simulink model "LAB07_1_copia2"  (R2022b)
settings: Solver=ode8  StartTime=0.0  StopTime=1000  FixedStep=0.1  RelTol=1e-3
values from neighbouring files (symbols this model uses):
  a = 6.843e6    (= 6843000)    [LAB_07_script.m]    (also in LAB_07_with3Dplot.m)
  A0 = eye(3,3)    [LAB_07_script.m]    (also in LAB_07_with3Dplot.m)
  A1 = 0.02    [LAB_07_with3Dplot.m]
  A2 = A1    (= 0.02)    [LAB_07_with3Dplot.m]
  A3 = A1    (= 0.02)    [LAB_07_with3Dplot.m]
  alpha_1 = 0.5    [LAB_07_with3Dplot.m]
  alpha_2 = 0.5    [LAB_07_with3Dplot.m]
  C_d = 2.1    [LAB_07_with3Dplot.m]
  e = 0    [LAB_07_script.m]    (also in LAB_07_with3Dplot.m)
  epsilon = 0.4093    [LAB_07_script.m]    (also in LAB_07_with3Dplot.m)
  G = 6.6743e-11    [LAB_07_script.m]    (also in LAB_07_with3Dplot.m)
  g_01 = -29404.8    [LAB_07_script.m]    (also in LAB_07_with3Dplot.m)
  g_11 = -1450.9    [LAB_07_script.m]    (also in LAB_07_with3Dplot.m)
  h_11 = 4652.5    [LAB_07_script.m]    (also in LAB_07_with3Dplot.m)
  i = 0.1    [LAB_07_script.m]    (also in LAB_07_with3Dplot.m)
  I = 10^-2*diag([100.9,25.1,91.6])    [LAB_07_script.m]    (also in LAB_07_with3Dplot.m)
  j_B = [0.01;0.05;0.01]    [LAB_07_script.m]    (also in LAB_07_with3Dplot.m)
  M_Earth = 5.972e24    (= 5.972e+24)    [LAB_07_script.m]    (also in LAB_07_with3Dplot.m)
  n = sqrt(G*M_Earth/a^3)    [LAB_07_script.m]    (also in LAB_07_with3Dplot.m)
  n_sun = 2*pi/T_sun    (= 1.99238499086e-07)    [LAB_07_script.m]    (also in LAB_07_with3Dplot.m)
  P = F_e/c    (= 4.52666666667e-06)    [LAB_07_script.m]    (also in LAB_07_with3Dplot.m)
  position = 1e-2*[10,0,0;0,10,0;-10,0,0;0,-10,0;0,0,15;                                     0,0,-15;0,45,0;0,45,0;0,-45,0;0,-45,0]    [LAB_07_script.m]    (also in LAB_07_with3Dplot.m)
  R_Earth = 6.378e6    (= 6378000)    [LAB_07_script.m]    (also in LAB_07_with3Dplot.m)
  R_sun = 149597870000    [LAB_07_script.m]    (also in LAB_07_with3Dplot.m)
  rhoD_vector = ones(10,1)*0.1    [LAB_07_script.m]    (also in LAB_07_with3Dplot.m)
  rhoS_vector = ones(10,1)*0.5    [LAB_07_script.m]    (also in LAB_07_with3Dplot.m)
  Surfaces_Matrix = [6e-2;6e-2;6e-2;6e-2;4e-2;4e-2;12e-2;                                                     12e-2;12e-2;12e-2]    [LAB_07_script.m]    (also in LAB_07_with3Dplot.m)
  theta0 = 0    [LAB_07_script.m]    (also in LAB_07_with3Dplot.m)
  Theta_m = deg2rad(11.5)    [LAB_07_script.m]    (also in LAB_07_with3Dplot.m)
  Versor_Surfaces_Matrix = [  1 , 0 ,-1 , 0 , 0 , 0 , 1 ,-1 , 1 ,-1 ... (first row only)    [LAB_07_script.m]    (also in LAB_07_with3Dplot.m)
  w0 = [0;0;0.01]    [LAB_07_script.m]    (also in LAB_07_with3Dplot.m = [1;1;1])
  w_Earth = 7.29e-5    (= 7.29e-05)    [LAB_07_script.m]    (also in LAB_07_with3Dplot.m)
undefined symbols (not defined in the file or in its folder): Gyroscope, HS, magnitude
libraries: simulink_extras x8, matrix_library x5, sharedutil x4, vrlib x3
(part 2 of 2)

== matlab function LAB07_1_copia2/Drag Perturbances/Air density relation ==
  data: r_N input; R_Earth input; rho output
function rho = density_calculator(r_N, R_Earth)
% Exponential model for computing density

h = (norm(r_N') - R_Earth)/1e+3;


H = 0;
h0 = 0;
rho_0 = 0; 

if h > 200 && h <= 250
    H = 38.5;
    h0 = 200;
    rho_0 = 2.780e-10;
elseif h > 250 && h <= 300
    H = 46.9;
    h0 = 250;
    rho_0 = 7.248e-11;
elseif h > 300 && h <= 350
    H = 52.5;
    h0 = 300;
    rho_0 = 2.418e-11;
elseif h > 350 && h <= 400
    H = 56.4;
    h0 = 350;
    rho_0 = 9.158e-12;
elseif h > 400 && h <= 450
    H = 59.4;
    h0 = 400;
    rho_0 = 3.725e-12;
elseif h > 450 && h <= 500
    H = 62.2;
    h0 = 450;
    rho_0 = 1.585e-12;
elseif h > 500 && h <= 600
    H = 65.8;
    h0 = 500;
    rho_0 = 6.967e-13;
elseif h > 600 && h <= 700
    H = 79.0;
    h0 = 600;
    rho_0 = 1.454e-13;
elseif h > 700 && h <= 800
    H = 109.0;
    h0 = 700;
    rho_0 = 3.614e-14;
elseif h > 800 && h <= 900
    H = 164.0;
    h0 = 800;
    rho_0 = 1.170e-14;
elseif h > 900 && h < 1000
    H = 225.0;
    h0 = 900;
    rho_0 = 5.245e-15;
elseif h > 1000 
    H = 260.0;
    h0 = 1000;
    rho_0 = 3.019e-15;
end

rho = rho_0*exp(-(h-h0)/H)*1e+20;
